simulink model "simulate_filter"  (R2015a)
settings: Solver=ode3  StartTime=0.0  StopTime=Tf  FixedStep=Ts  RelTol=1e-3
values from neighbouring files (symbols this model uses):
  A = 0.35    [ECE310main.m]    (also in ECE341P6_6.m = i*(w*ur*uo))
  B = complex(sigma, w*er*eo)    [ECE341P6_6.m]
  Ts = 1/R    (= 0.0002)    [ECE310main.m]    (also in check_filter.m = t(2)-t(1); test_filters.m = t(2)-t(1); wheel_parameters.m = 0.05)
settings Model: Creator=throne  LastModifiedBy=throne

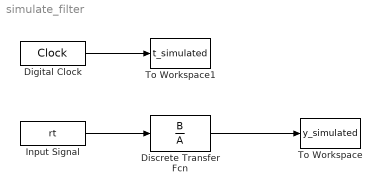
== system simulate_filter ==
  Digital Clock : DigitalClock  SampleTime=Ts
  Discrete Transfer Fcn : DiscreteTransferFcn  Numerator=B  Denominator=A  SampleTime=Ts
  "Input Signal " : FromWorkspace  VariableName=rt  SampleTime=Ts
  To Workspace : ToWorkspace  VariableName=y_simulated  SampleTime=-1
  To Workspace1 : ToWorkspace  VariableName=t_simulated  SampleTime=-1
  wires:
  Discrete Transfer Fcn/1 -> To Workspace/1
  "Input Signal "/1 -> Discrete Transfer Fcn/1
  Digital Clock/1 -> To Workspace1/1
